simulink model "AllObserverComparisonTest1"  (R2019b)
settings: Solver=FixedStepAuto  StartTime=0.0  StopTime=timeStop  FixedStep=timeStep  RelTol=1e-3
values from neighbouring files (symbols this model uses):
  b20 = 40    [paraSetting.m]
  focalLen = 20    [paraSetting.m]
  k123 = 0.12    [paraSetting.m]
  lamda5 = 0.15    [paraSetting.m]
  M9 = 0.03    [paraSetting.m]
  modelSelection = 4    [paraSetting.m]
  rou20 = 0.018    [paraSetting.m]
settings Model: PauseTimes=1.3  Creator=lixiangfei  LastModifiedBy=lixiangfei
settings DataIOCC: ReturnWorkspaceOutputs=off
settings DebuggingCC: ArithmeticOperatorsInVariantConditions=warning
settings SFSimCC: SimUseLocalCustomCode=off  CustomCodeUndefinedFunction=UseInterfaceOnly
settings RTWCC: RTWUseLocalCustomCode=off

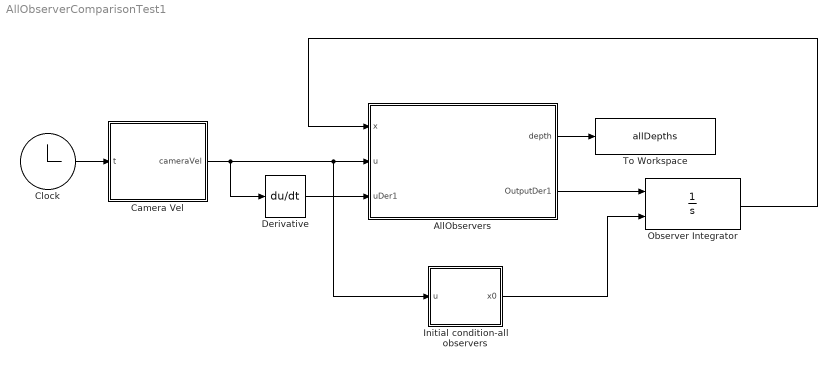
== system AllObserverComparisonTest1 ==
  AllObservers : MATLAB Function  TreatAsAtomicUnit=on
  Camera Vel : MATLAB Function  TreatAsAtomicUnit=on
  Clock : Clock
      settings: Decimation=5
  Derivative : Derivative
  Initial condition-all observers : MATLAB Function  TreatAsAtomicUnit=on
  Observer Integrator : Integrator  InitialConditionSource=external  InitialCondition=[10, 5, 2, 10, 5, 5, -2.2734]
  To Workspace : ToWorkspace  VariableName=allDepths  SaveFormat=Structure With Time  SampleTime=-1
  wires:
  Clock/1 -> Camera Vel/1(t)
  AllObservers/2(OutputDer1) -> Observer Integrator/1
  Observer Integrator/1 -> AllObservers/1(x)
  Camera Vel/1(cameraVel) -> AllObservers/2(u), Initial condition-all observers/1(u), Derivative/1
  Initial condition-all observers/1(x0) -> Observer Integrator/2
  AllObservers/1(depth) -> To Workspace/1
  Derivative/1 -> AllObservers/3(uDer1)

== matlab function AllObserverComparisonTest1/Camera Vel ==
  settings: updateMethod=DISCRETE
  data: t input; cameraVel output; modelSelection parameter
function cameraVel = Model(t,modelSelection)
%% 设置相机速度
cameraVel = zeros(1,6);

% 选择对应的相机速度
if modelSelection == 1
    % 该速度用于验证全局收敛性
    cameraVel(1) = 0.1;
    cameraVel(2) = 0.2;
    cameraVel(3) = -0.8;
    cameraVel(4) = sin(pi*t);
    cameraVel(5) = pi/15;
    cameraVel(6) = pi/8;      
end

== matlab function AllObserverComparisonTest1/AllObservers ==
  settings: updateMethod=DISCRETE
  data: depth output; x input; u input; OutputDer1 output; uDer1 input; focalLen parameter; lamda5 parameter; M9 parameter; k123 parameter; rou20 parameter; b20 parameter
function [depth, OutputDer1] = Observer(x, u, uDer1, focalLen, lamda5, M9, k123, rou20, b20)
%% 模型初始化
% 初始化输出
depth = zeros(1, 5);
OutputDer1 = zeros(1,7);

% 系统动力学
OutputDer1(1:3) = [-focalLen*x(3), 0, x(1)*x(3), x(1)*x(2)/focalLen, -(focalLen+x(1)^2/focalLen), x(2);
          0, -focalLen*x(3), x(2)*x(3), (focalLen+x(2)^2/focalLen), -x(1)*x(2)/focalLen, -x(1);
          0, 0, x(3)^2, x(2)*x(3)/focalLen, -x(1)*x(3)/focalLen, 0] * u';
% 未加噪声
temp = [x(1), x(2)];

%% A New solution to the Problem of Range Identification In  Perspective Vision Systems
% 2005 IEEE AC; Author:  Dimitrios Karagiannis et al. 
% 观测器模型
y5 = temp;
eitaHat5 = x(4);
beita5 = 0.5*lamda5*((y5(1)^2 + y5(2)^2)*u(3) - 2*u(1)*y5(1)*focalLen - 2*u(2)*y5(2)*focalLen);
beita5Der1y = [lamda5*(-u(1)*focalLen + u(3)*y5(1)), lamda5*(-u(2)*focalLen + u(3)*y5(2))];
beita5Der1t = 0.5*lamda5*((y5(1)^2 + y5(2)^2)*uDer1(3) - 2*uDer1(1)*y5(1)*focalLen - 2*uDer1(2)*y5(2)*focalLen);

p51yt = [y5(1)*y5(2)*u(4)/focalLen - (focalLen+y5(1)^2/focalLen)*u(5) + y5(2)*u(6); (focalLen+y5(2)^2/focalLen)*u(4) - y5(1)*y5(2)*u(5)/focalLen - y5(1)*u(6)];
p52yt = (y5(2)*u(4) - y5(1)*u(5))/focalLen;
g5yt = [-focalLen*u(1) + y5(1)*u(3); -focalLen*u(2) + y5(2)*u(3)];

% 观测器输出
OutputDer1(4) = p52yt * (eitaHat5 + beita5) + u(3)*(eitaHat5 + beita5)^2 - beita5Der1t...
    - beita5Der1y * ( p51yt + g5yt * (eitaHat5 + beita5));
            
%% Range estimation from a moving camera: an Immersion and Invariance approach
% 2009 ICRA; Author:  Fabio Morbidi et al.
y9 = temp;
p91yt = [y9(1)*y9(2)*u(4)/focalLen - (focalLen+y9(1)^2/focalLen)*u(5) + y9(2)*u(6); (focalLen+y9(2)^2/focalLen)*u(4) - y9(1)*y9(2)*u(5)/focalLen - y9(1)*u(6)];
p92yt = (y9(2)*u(4) - y9(1)*u(5))/focalLen;
g9yt = [-focalLen*u(1) + y9(1)*u(3); -focalLen*u(2) + y9(2)*u(3)];

% 观测器输出
eitaHat9 = (0.5*M9*(u(3)*(y9(1)^2 + y9(2)^2) - 2 * focalLen * (u(1)*y9(1) + u(2)*y9(2))) - x(5))*norm(g9yt);
OutputDer1(5) = M9 * g9yt'*(p91yt + eitaHat9 * g9yt) - ...
    0.5*M9*(-uDer1(3)*(y9(1)^2 + y9(2)^2) + 2 * focalLen * (uDer1(1)*y9(1)+uDer1(2)*y9(2))) - (p92yt*eitaHat9+u(3)*eitaHat9^2)/norm(g9yt) + ...
    eitaHat9/(norm(g9yt))^3 * g9yt'* (u(3)*(p91yt + eitaHat9 * g9yt) + [-focalLen * uDer1(1) + y9(1)*uDer1(3); -focalLen * uDer1(2) + y9(2)*uDer1(3)]);

%% Globally exponentially stable observer for vision-based range estimation
% 2012 Mechatronics; Author: A.P. Dani et al.
y12 = temp;

% 计算辅助状态变量
b121 = -u(1);
b122 = -u(2);
b123 = -u(3);
w121 = -u(4);
w122 = -u(5);
w123 = -u(6);
b121Der1 = -uDer1(1);
b122Der1 = -uDer1(2);
b123Der1 = -uDer1(3);
aerfa12 = x(6);

% 计算beta值
beta12 = k123*(b121*y12(1)*focalLen + b122*y12(2)*focalLen - b123*(0.5*(y12(1)^2 + y12(2)^2)));

% 计算中间变量
h121 = focalLen*b121 - y12(1)*b123;
h122 = focalLen*b122 - y12(2)*b123;
p121 = -y12(1)*y12(2)*w121/focalLen + (focalLen+y12(1)^2/focalLen)*w122 - y12(2)*w123;
p122 = -(focalLen+y12(2)^2/focalLen)*w121 + y12(1)*y12(2)*w122/focalLen + y12(1)*w123;
p123 = (y12(2)*w121 - y12(1)*w122)/focalLen;

% 观测器的输出 
OutputDer1(6) = (aerfa12 + beta12)^2*b123 + p123*(aerfa12 + beta12)-k123*(h121^2+h122^2)*(aerfa12 + beta12)-k123*h121*p121 -....
    k123*h122*p122 - k123*y12(1)*b121Der1*focalLen-k123*y12(2)*b122Der1*focalLen + k123*b123Der1*(0.5*(y12(1)^2+y12(2)^2));

%% Proposed observer
% 2020 ; Author: Xiangfei Li et al.
y20 = temp;
eitaHat20 = x(7);

% 观测器模型
fai20 = - u(1)*y20(1)*focalLen - u(2)*y20(2)*focalLen + 0.5*u(3)*y20(1)^2 + 0.5*u(3)*y20(2)^2;
fai20Der1y = [-u(1)*focalLen + u(3)*y20(1), -u(2)*focalLen + u(3)*y20(2)];
fai20Der1t = 0.5*(y20(1)^2 + y20(2)^2)*uDer1(3) - uDer1(1)*y20(1)*focalLen - uDer1(2)*y20(2)*focalLen;

p201yt = [y20(1)*y20(2)*u(4)/focalLen - (focalLen+y20(1)^2/focalLen)*u(5) + y20(2)*u(6); (focalLen+y20(2)^2/focalLen)*u(4) - y20(1)*y20(2)*u(5)/focalLen - y20(1)*u(6)];
p202yt = (y20(2)*u(4) - y20(1)*u(5))/focalLen;
g20yt = [-focalLen*u(1) + y20(1)*u(3); -focalLen*u(2) + y20(2)*u(3)];

% 观测器输出
OutputDer1(7) = p202yt/log(b20) - rou20* (fai20Der1y * p201yt + fai20Der1t) - (b20^(eitaHat20 + rou20*fai20))*(-u(3)/log(b20) + rou20 * fai20Der1y * g20yt);

%% 输出深度值
% 模型的真实值
state = x;
depth(1) = 1/state(3);

% 2005 A New solution to the Problem of Range Identification In  Perspective Vision Systems
y5 = temp;
beita5 = 0.5*lamda5*((y5(1)^2 + y5(2)^2)*u(3) - 2*u(1)*y5(1)*focalLen - 2*u(2)*y5(2)*focalLen);
depth(2) = 1/(state(4) + beita5);

% 2009 Range estimation from a moving camera: an Immersion and Invariance approach
y9 = temp;
g9yt = [-focalLen*u(1) + y9(1)*u(3); -focalLen*u(2) + y9(2)*u(3)];

depth(3) = 1/((0.5*M9*(u(3)*(y9(1)^2 + y9(2)^2) - 2 * focalLen * (u(1)*y9(1) + u(2)*y9(2))) - state(5))*norm(g9yt));

% 2012 Globally exponentially stable observer for vision-based range estimation
y12 = temp;
beta12 = k123*(b121*y12(1)*focalLen + b122*y12(2)*focalLen - b123*(0.5*(y12(1)^2 + y12(2)^2)));

depth(4) = 1/(state(6) + beta12);

% 2020 Proposed observer
y20 = temp;
fai20 = - u(1)*y20(1)*focalLen - u(2)*y20(2)*focalLen + 0.5*u(3)*y20(1)^2 + 0.5*u(3)*y20(2)^2;
depth(5) = 1/b20^(state(7) + rou20 * fai20);
end

== matlab function AllObserverComparisonTest1/Initial condition-all observers ==
  data: x0 output; u input; focalLen parameter; modelSelection parameter; lamda5 parameter; M9 parameter; k123 parameter; rou20 parameter; b20 parameter
function x0 = initialValue(u, focalLen, modelSelection, lamda5, M9, k123, rou20, b20)
%% 选择不同模型
x0 = zeros(1,7);
    
if modelSelection == 1
    % 设置系统动力学真实的初值
    x0(1) = 3;
    x0(2) = 1.5;
    x0(3) = 0.25;

    % 设置观测器初始值的差值
    errorValue = 3.96;

    % 设置各观测器初始值
    % A New solution to the Problem of Range Identification In  Perspective Vision Systems
    % 2005 IEEE AC; Author:  Dimitrios Karagiannis et al. 
    y5 = [x0(1), x0(2)]';
    beita5Initial = 0.5*lamda5*((y5(1)^2 + y5(2)^2)*u(3) - 2*u(1)*y5(1)*focalLen - 2*u(2)*y5(2)*focalLen);
    x0(4) = 1/(1/x0(3)-errorValue) - beita5Initial;

    % Range estimation from a moving camera: an Immersion and Invariance approach
    % 2009 ICRA; Author:  Fabio Morbidi et al.
    y9 = [x0(1), x0(2)]';
    g9yt = [-focalLen*u(1) + y9(1)*u(3); -focalLen*u(2) + y9(2)*u(3)];
    
    x0(5) = -(1/(1/x0(3) - errorValue))/norm(g9yt) + 0.5*M9*(u(3)*(y9(1)^2 + y9(2)^2) - 2 * focalLen * (u(1)*y9(1) + u(2)*y9(2)));
    
    % Globally exponentially stable observer for vision-based range estimation
    % 2012 Mechatronics; Author: A.P. Dani et al.
    y12 = [x0(1), x0(2)]';
    beita12Initial = k123*(-u(1)*y12(1)*focalLen - u(2)*y12(2)*focalLen + u(3)*(0.5*(y12(1)^2 + y12(2)^2)));

    x0(6) = 1/(1/x0(3)-errorValue) - beita12Initial;    

    % 2020 Proposed observer
    y20 = [x0(1), x0(2)]';

    fai20 = - u(1)*y20(1)*focalLen - u(2)*y20(2)*focalLen + 0.5*u(3)*y20(1)^2 + 0.5*u(3)*y20(2)^2;
    x0(7) = log(1/(1/x0(3) - errorValue))/log(b20) - rou20 * fai20;
    x0;    
end
end
